simulink model "gm_DirectForm_2016a"  (R2016a)
settings: Solver=VariableStepAuto  StartTime=0.0  StopTime=10.0  RelTol=1e-3
settings Model: Creator=Arthur  LastModifiedBy=Arthur
settings OptimizationCC: BlockReduction=off  ConditionallyExecuteInputs=off
settings DebuggingCC: InheritedTsInSrcMsg=none

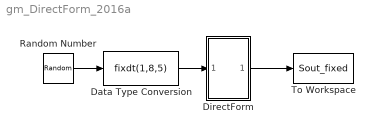
== system gm_DirectForm_2016a ==
  Data Type Conversion : DataTypeConversion  OutDataTypeStr=fixdt(1,8,5)
  DirectForm : Subsystem
  Random Number : RandomNumber  SampleTime=0.1
  To Workspace : ToWorkspace  VariableName=Sout_fixed  SaveFormat=Timeseries  SampleTime=-1
  wires:
  Data Type Conversion/1 -> DirectForm/1(In1)
  DirectForm/1(Out1) -> To Workspace/1
  Random Number/1 -> Data Type Conversion/1

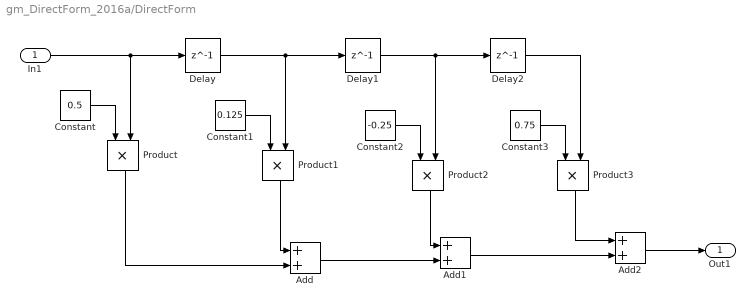
== system gm_DirectForm_2016a/DirectForm ==
  In1 : Inport
  Add : Sum  OutDataTypeStr=fixdt(1,8,6)
  Add1 : Sum  OutDataTypeStr=fixdt(1,8,6)
  Add2 : Sum  OutDataTypeStr=fixdt(1,8,5)
  Constant : Constant  Value=0.5  OutDataTypeStr=fixdt(0,1,1)
  Constant1 : Constant  Value=0.125  OutDataTypeStr=fixdt(0,3,3)
  Constant2 : Constant  Value=-0.25  OutDataTypeStr=fixdt(1,3,2)
  Constant3 : Constant  Value=0.75  OutDataTypeStr=fixdt(0,2,2)
  Delay : Delay  DelayLength=1
  Delay1 : Delay  DelayLength=1
  Delay2 : Delay  DelayLength=1
  Product : Product  OutDataTypeStr=fixdt(1,8,6)
  Product1 : Product  OutDataTypeStr=fixdt(1,8,7)
  Product2 : Product  OutDataTypeStr=fixdt(1,8,7)
  Product3 : Product  OutDataTypeStr=fixdt(1,8,6)
  Out1 : Outport
  wires:
  Constant/1 -> Product/1
  Constant3/1 -> Product3/1
  In1/1 -> Delay/1, Product/2
  Add/1 -> Add1/2
  Constant2/1 -> Product2/1
  Product3/1 -> Add2/1
  Add1/1 -> Add2/2
  Product2/1 -> Add1/1
  Constant1/1 -> Product1/1
  Delay1/1 -> Delay2/1, Product2/2
  Product1/1 -> Add/1
  Product/1 -> Add/2
  Delay/1 -> Product1/2, Delay1/1
  Add2/1 -> Out1/1
  Delay2/1 -> Product3/2
